simulink model "IEEE123_4subsystem"  (R2022b)
settings: Solver=ode4  StartTime=0.0  StopTime=inf  FixedStep=Ts  MaxStep=1e-4  RelTol=1e-3
PreLoadFcn:
  | Ts = 50e-6;
PostLoadFcn:
  | Ts = 50e-6;
InitFcn:
  | %%%%%%%%%%%%%%%%%%%%%%%%
  | % Simulation data for the IEEE 123 Node Test Feeder model
  | %%%%%%%%%%%%%%%%%%%%%%%
  | 
  | % miles/km
  | mi2km = 1.60934;
  | 
  | % feet to km
  | ft2km = 0.0003048;
  | 
  | % microsiemens to Farads
  | ms2F = 1/2/pi/60*1e-6;
  | 
  | %% Configuration 1 - series reactance - ohm/mile
  | 
  | R_1 = [0.4576 0.1560 0.1535;0.1560 0.4666 0.1580;0.1535 0.1580 0.4615];
  | X_1 = [1.0780 0.5017 0.3849;0.5017 1.0482 0.4236;0.3849 0.4236 1.0651];
  | 
  | % charging susceptance - microsiemens/mile
  | 
  | B_1 = [5.6765 -1.8319 -0.6982;-1.8319 5.9809 -1.1645;-0.6982 -1.1645 5.3971];
  | 
  | % convert for SPS
  | 
  | R_1 = R_1/mi2km;
  | 
  | Rs_1=(R_1(1,1)+R_1(2,2)+R_1(3,3))/3;
  | Rm_1=(R_1(1,2)+R_1(1,3)+R_1(2,3))/3;
  | R1_1=Rs_1-Rm_1;
  | R0_1=Rs_1+2*Rm_1;
  | 
  | L_1 = X_1/mi2km/2/pi/60;
  | 
  | Ls_1=(L_1(1,1)+L_1(2,2)+L_1(3,3))/3;
  | Lm_1=(L_1(1,2)+L_1(1,3)+L_1(2,3))/3;
  | L1_1=Ls_1-Lm_1;
  | L0_1=Ls_1+2*Lm_1;
  | 
  | C_1 = B_1/mi2km*ms2F;
  | 
  | Cs_1=(C_1(1,1)+C_1(2,2)+C_1(3,3))/3;
  | Cm_1=(C_1(1,2)+C_1(1,3)+C_1(2,3))/3;
  | C1_1=Cs_1-Cm_1;
  | C0_1=Cs_1+2*Cm_1;
  | 
  | 
  | %% Configuration 2 - series reactance - ohm/mile
  | 
  | R_2 = [0.4666 0.1580 0.1560;0.1580 0.4615 0.1535;0.1560 0.1535 0.4576];
  | X_2 = [1.0482 0.4236 0.5017;0.4236 1.0651 0.3849;0.5017 0.3849 1.0780];
  | 
  | % charging susceptance - microsiemens/mile
  | 
  | B_2 = [5.9809 -1.1645 -1.8319;-1.1645 5.3971 -0.6982;-1.8319 -0.6982 5.6765];
  | 
  | % convert for SPS
  | 
  | R_2 = R_2/mi2km;
  | 
  | Rs_2=(R_2(1,1)+R_2(2,2)+R_2(3,3))/3;
  | ... (+341 lines)
undefined symbols (not defined in the file): D1, Delta, find_system, I, Left, MOV_segment9, powergui, Right, type, V, X
libraries: spsGroundLib x242, spsThreePhaseVIMeasurementLib x134, spsSeriesRLCBranchLib x107, spsSeriesRLCLoadLib x83, spsPiSectionLineLib x61, spsThreePhasePISectionLineLib x60, spsVoltageMeasurementLib x52, spsDCVoltageSourceLib x36, ssn_lib x28, artemis x24, spsACCurrentSourceLib x18, spsOnDelayLib x18
(part 8 of 15)

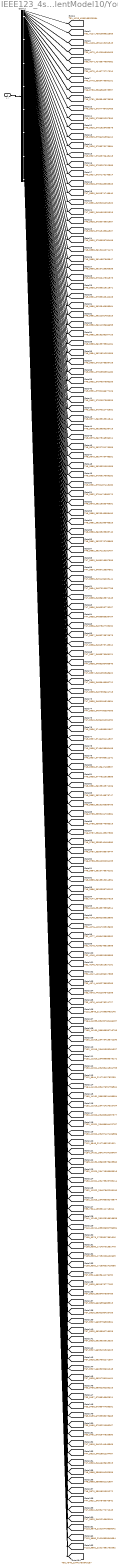
== system IEEE123_4subsystem/powergui/EquivalentModel10/Yout ==
  v,i : Inport
  Demux : Demux  Outputs=[1 1 1 1 1 1 1 1 1 1 1 1 1 1 1 1 1 1 1 1 1 1 1 1 1 1 1 1 1 1 1 1 1 1 1 1 1 1 1 1 1 1 1 1 1 1 1 1 1 1 1 1 1 1 1 1 1 1 1 1 1 1 1 1 1 1 1 1 1 1 1 1 1 1 1 1 1 1 1 1 1 1 1 1 1 1 1 1 1 1 1 1 1 1 1 1 1 1 1 1 1 1 1 1 1 1 1 1 1 1 1 1 1 1 1 1 1 1 1 1 1 1 1 1 1 1 1 1 1 1 1 1 1 1 1 1 1 1 1 1 1 1 1 1 1 1 1 1 1 1 1 1 1 1 1 1 1 1 1 1 1 1 1 1]
  tag scope: T109_9379_17239517861616=global, T109_9380_17245701551478=global, T109_9381_17252206402625=global, T109_9382_17259032415056=global, T112_9843_21170965463146=global, T112_9844_21171312782239=global, T112_9845_21171852131511=global, T113_9879_21016479838042=global, T113_9880_21016835649654=global, T113_9881_21017381792062=global, T132_11318_25473415572290=global, T132_11319_25472424310754=global, T132_11319_25481353264337=global, T132_11320_25471595983916=global, T132_11320_25480360057377=global, T132_11320_25489689575172=global, T132_11321_25479529785114=global, T132_11321_25488694422787=global, T132_11321_25498424504795=global, T132_11322_25487862205100=global, T132_11322_25497427406986=global, T132_11323_25496593243874=global, T141_12160_28102518618639=global, T142_12211_28300682796084=global, T164_14099_38430760466187=global, T164_14100_38427691756561=global, T164_14101_38424754189497=global, T165_14150_38606899716706=global, T165_14151_38603824498954=global, T165_14152_38600879628960=global, T46_3779_3365479900101=global, T46_3780_3366960378957=global, T46_3781_3368545675638=global, T46_3785_3359104702884=global, T46_3786_3358240484580=global, T46_3786_3360574906319=global, T46_3787_3359708975444=global, T46_3787_3362149927580=global, T46_3788_3361282284135=global, T47_3818_3461244945569=global, T47_3819_3462881234487=global, T47_3820_3464625615319=global, T47_3821_3457845970842=global, T47_3822_3459477271045=global, T47_3823_3461216663164=global, T47_3830_3491574748640=global, T47_3831_3493184294320=global, T47_3832_3494901931915=global, T47_3833_3488118997595=global, T47_3834_3487013057798=global, T47_3834_3489723554561=global, T47_3835_3485966639704=global, T47_3835_3488615871045=global, T47_3835_3491436203441=global, T47_3836_3484979743312=global, T47_3836_3487567709232=global, T47_3836_3490326776207=global, T47_3837_3484052368622=global, T47_3837_3486579069121=global, T47_3837_3489276870675=global, T47_3838_3483184515634=global, T47_3838_3485649950712=global, T47_3838_3488286486846=global, T47_3839_3484780354006=global, T47_3839_3487355624718=global, T47_3840_3486484284292=global, T48_3868_3588184282939=global, T48_3869_3589952131897=global, T48_3870_3591831351272=global, T48_3877_3623913311844=global, T48_3878_3622731176059=global, T48_3878_3625659238719=global, T48_3879_3621603340691=global, T48_3879_3624475448351=global, T48_3879_3627516536011=global, T48_3880_3620529805740=global, T48_3880_3620540608364=global, T48_3880_3623345958400=global, T48_3880_3626331091059=global, T48_3881_3619510571206=global, T48_3881_3622270768865=global, T48_3881_3622281452323=global, T48_3881_3625199946525=global, T48_3882_3618238287726=global, T48_3882_3621249879747=global, T48_3882_3624123102407=global, T48_3882_3624133666698=global, T48_3883_3619975584184=global, T48_3883_3623100558706=global, T48_3884_3616778670102=global, T48_3884_3621824251059=global, T48_3885_3618513014894=global, T48_3886_3620358730102=global, T48_3888_3613161071472=global, T48_3889_3614887665847=global, T48_3890_3616725630638=global, T49_3924_3757748792483=global, T49_3925_3756494356412=global, T49_3925_3759631297500=global, T49_3926_3755297012585=global, T49_3926_3758375175884=global, T49_3926_3761628455578=global, T49_3927_3757176146514=global, T49_3927_3760370648418=global, T49_3928_3753073601667=global, T49_3928_3759169933503=global, T49_3929_3752047534575=global, T49_3929_3754949364507=global, T49_3930_3750614909252=global, T49_3930_3751078559728=global, T49_3930_3753921611871=global, T49_3930_3756939780408=global, T49_3931_3750166677126=global, T49_3931_3752487418180=global, T49_3931_3752950951480=global, T49_3931_3755910342228=global, T49_3932_3752037383333=global, T49_3932_3754474580170=global, T49_3932_3754937996293=global, T49_3933_3754022742602=global, T49_3936_3744588901667=global, T49_3937_3743786611241=global, T49_3937_3746451414507=global, T49_3938_3745647438537=global, T49_3938_3748428580408=global, T49_3939_3747622918895=global, T50_4073_4242094590453=global, T50_4074_4243874684082=global, T50_4075_4245772717310=global, T50_4147_3946663207629=global, T50_4148_3948375596914=global, T50_4149_3950205925800=global, T51_4126_4390185320384=global, T51_4127_4392089622565=global, T51_4128_4394115154549=global, T51_4276_4184720319600=global, T51_4277_4186423803302=global, T51_4278_4188248516808=global, T52_4245_4199931959955=global, T52_4246_4201921827191=global, T52_4247_4204036217888=global, T53_4374_4430278693266=global, T53_4375_4432264542308=global, T53_4376_4434378211727=global, T63_5456_6800230253216=global, T63_5457_6799516962811=global, T63_5458_6798947459391=global, T63_5459_6793938078669=global, T63_5460_6793221056267=global, T63_5461_6792647820850=global, T67_5524_6628644176192=global, T67_5525_6626590718028=global, T67_5525_6626956688313=global, T67_5525_6631975777182=global, T67_5526_6624902271307=global, T67_5526_6629920913320=global, T67_5526_6630286426753=global, T67_5526_6635487595785=global, T67_5527_6628230604048=global, T67_5527_6633431326223=global, T67_5527_6633796382804=global, T67_5528_6631739154401=global, T89_7904_13533111748011=global, T90_7940_13442750943157=global
  wires:
  v,i/1 -> Demux/1
  Demux/1 -> [T51_4126_4390185320384]
  Demux/2 -> [T51_4127_4392089622565]
  Demux/3 -> [T51_4128_4394115154549]
  Demux/4 -> [T50_4073_4242094590453]
  Demux/5 -> [T50_4074_4243874684082]
  Demux/6 -> [T50_4075_4245772717310]
  Demux/7 -> [T46_3779_3365479900101]
  Demux/8 -> [T46_3780_3366960378957]
  Demux/9 -> [T46_3781_3368545675638]
  Demux/10 -> [T49_3924_3757748792483]
  Demux/11 -> [T49_3925_3759631297500]
  Demux/12 -> [T49_3926_3761628455578]
  Demux/13 -> [T49_3925_3756494356412]
  Demux/14 -> [T49_3926_3758375175884]
  Demux/15 -> [T49_3927_3760370648418]
  Demux/16 -> [T49_3926_3755297012585]
  Demux/17 -> [T49_3927_3757176146514]
  Demux/18 -> [T49_3928_3759169933503]
  Demux/19 -> [T47_3830_3491574748640]
  Demux/20 -> [T47_3831_3493184294320]
  Demux/21 -> [T47_3832_3494901931915]
  Demux/22 -> [T49_3928_3753073601667]
  Demux/23 -> [T49_3929_3754949364507]
  Demux/24 -> [T49_3930_3756939780408]
  Demux/25 -> [T48_3888_3613161071472]
  Demux/26 -> [T48_3889_3614887665847]
  Demux/27 -> [T48_3890_3616725630638]
  Demux/28 -> [T49_3929_3752047534575]
  Demux/29 -> [T49_3930_3753921611871]
  Demux/30 -> [T49_3931_3755910342228]
  Demux/31 -> [T48_3880_3620540608364]
  Demux/32 -> [T48_3881_3622281452323]
  Demux/33 -> [T48_3882_3624133666698]
  Demux/34 -> [T48_3882_3618238287726]
  Demux/35 -> [T48_3883_3619975584184]
  Demux/36 -> [T48_3884_3621824251059]
  Demux/37 -> [T49_3930_3751078559728]
  Demux/38 -> [T49_3931_3752950951480]
  Demux/39 -> [T49_3932_3754937996293]
  Demux/40 -> [T49_3931_3750166677126]
  Demux/41 -> [T49_3932_3752037383333]
  Demux/42 -> [T49_3933_3754022742602]
  Demux/43 -> [T48_3877_3623913311844]
  Demux/44 -> [T48_3878_3625659238719]
  Demux/45 -> [T48_3879_3627516536011]
  Demux/46 -> [T48_3878_3622731176059]
  Demux/47 -> [T48_3879_3624475448351]
  Demux/48 -> [T48_3880_3626331091059]
  Demux/49 -> [T49_3930_3750614909252]
  Demux/50 -> [T49_3931_3752487418180]
  Demux/51 -> [T49_3932_3754474580170]
  Demux/52 -> [T48_3879_3621603340691]
  Demux/53 -> [T48_3880_3623345958400]
  Demux/54 -> [T48_3881_3625199946525]
  Demux/55 -> [T48_3880_3620529805740]
  Demux/56 -> [T48_3881_3622270768865]
  Demux/57 -> [T48_3882_3624123102407]
  Demux/58 -> [T47_3833_3488118997595]
  Demux/59 -> [T47_3834_3489723554561]
  Demux/60 -> [T47_3835_3491436203441]
  Demux/61 -> [T47_3834_3487013057798]
  Demux/62 -> [T47_3835_3488615871045]
  Demux/63 -> [T47_3836_3490326776207]
  Demux/64 -> [T47_3835_3485966639704]
  Demux/65 -> [T47_3836_3487567709232]
  Demux/66 -> [T47_3837_3489276870675]
  Demux/67 -> [T47_3836_3484979743312]
  Demux/68 -> [T47_3837_3486579069121]
  Demux/69 -> [T47_3838_3488286486846]
  Demux/70 -> [T47_3837_3484052368622]
  Demux/71 -> [T47_3838_3485649950712]
  Demux/72 -> [T47_3839_3487355624718]
  Demux/73 -> [T47_3838_3483184515634]
  Demux/74 -> [T47_3839_3484780354006]
  Demux/75 -> [T47_3840_3486484284292]
  Demux/76 -> [T49_3936_3744588901667]
  Demux/77 -> [T49_3937_3746451414507]
  Demux/78 -> [T49_3938_3748428580408]
  Demux/79 -> [T49_3937_3743786611241]
  Demux/80 -> [T49_3938_3745647438537]
  Demux/81 -> [T49_3939_3747622918895]
  Demux/82 -> [T48_3881_3619510571206]
  Demux/83 -> [T48_3882_3621249879747]
  Demux/84 -> [T48_3883_3623100558706]
  Demux/85 -> [T46_3785_3359104702884]
  Demux/86 -> [T46_3786_3360574906319]
  Demux/87 -> [T46_3787_3362149927580]
  Demux/88 -> [T46_3786_3358240484580]
  Demux/89 -> [T46_3787_3359708975444]
  Demux/90 -> [T46_3788_3361282284135]
  Demux/91 -> [T48_3884_3616778670102]
  Demux/92 -> [T48_3885_3618513014894]
  Demux/93 -> [T48_3886_3620358730102]
  Demux/94 -> [T50_4147_3946663207629]
  Demux/95 -> [T50_4148_3948375596914]
  Demux/96 -> [T50_4149_3950205925800]
  Demux/97 -> [T51_4276_4184720319600]
  Demux/98 -> [T51_4277_4186423803302]
  Demux/99 -> [T51_4278_4188248516808]
  Demux/100 -> [T52_4245_4199931959955]
  Demux/101 -> [T52_4246_4201921827191]
  Demux/102 -> [T52_4247_4204036217888]
  Demux/103 -> [T53_4374_4430278693266]
  Demux/104 -> [T53_4375_4432264542308]
  Demux/105 -> [T53_4376_4434378211727]
  Demux/106 -> [T112_9843_21170965463146]
  Demux/107 -> [T164_14099_38430760466187]
  Demux/108 -> [T165_14150_38606899716706]
  Demux/109 -> [T132_11318_25473415572290]
  Demux/110 -> [T132_11319_25481353264337]
  Demux/111 -> [T132_11320_25489689575172]
  Demux/112 -> [T132_11321_25498424504795]
  Demux/113 -> [T112_9844_21171312782239]
  Demux/114 -> [T164_14100_38427691756561]
  Demux/115 -> [T165_14151_38603824498954]
  Demux/116 -> [T132_11319_25472424310754]
  Demux/117 -> [T132_11320_25480360057377]
  Demux/118 -> [T132_11321_25488694422787]
  Demux/119 -> [T132_11322_25497427406986]
  Demux/120 -> [T112_9845_21171852131511]
  Demux/121 -> [T164_14101_38424754189497]
  Demux/122 -> [T165_14152_38600879628960]
  Demux/123 -> [T132_11320_25471595983916]
  Demux/124 -> [T132_11321_25479529785114]
  Demux/125 -> [T132_11322_25487862205100]
  Demux/126 -> [T132_11323_25496593243874]
  Demux/127 -> [T89_7904_13533111748011]
  Demux/128 -> [T141_12160_28102518618639]
  Demux/129 -> [T142_12211_28300682796084]
  Demux/130 -> [T109_9379_17239517861616]
  Demux/131 -> [T109_9380_17245701551478]
  Demux/132 -> [T109_9381_17252206402625]
  Demux/133 -> [T109_9382_17259032415056]
  Demux/134 -> [T67_5524_6628644176192]
  Demux/135 -> [T67_5525_6631975777182]
  Demux/136 -> [T67_5526_6635487595785]
  Demux/137 -> [T67_5525_6626956688313]
  Demux/138 -> [T67_5526_6630286426753]
  Demux/139 -> [T67_5527_6633796382804]
  Demux/140 -> [T67_5525_6626590718028]
  Demux/141 -> [T67_5526_6629920913320]
  Demux/142 -> [T67_5527_6633431326223]
  Demux/143 -> [T67_5526_6624902271307]
  Demux/144 -> [T67_5527_6628230604048]
  Demux/145 -> [T67_5528_6631739154401]
  Demux/146 -> [T63_5456_6800230253216]
  Demux/147 -> [T63_5457_6799516962811]
  Demux/148 -> [T63_5458_6798947459391]
  Demux/149 -> [T63_5459_6793938078669]
  Demux/150 -> [T63_5460_6793221056267]
  Demux/151 -> [T63_5461_6792647820850]
  Demux/152 -> [T47_3818_3461244945569]
  Demux/153 -> [T47_3819_3462881234487]
  Demux/154 -> [T47_3820_3464625615319]
  Demux/155 -> [T48_3868_3588184282939]
  Demux/156 -> [T48_3869_3589952131897]
  Demux/157 -> [T48_3870_3591831351272]
  Demux/158 -> [T47_3821_3457845970842]
  Demux/159 -> [T47_3822_3459477271045]
  Demux/160 -> [T47_3823_3461216663164]
  Demux/161 -> [T113_9879_21016479838042]
  Demux/162 -> [T113_9880_21016835649654]
  Demux/163 -> [T113_9881_21017381792062]
  Demux/164 -> [T90_7940_13442750943157]

== system IEEE123_4subsystem/powergui/EquivalentModel11/Gates ==
  Mux : Mux  Inputs=[1 1 1 1 1 1 1 1 1]
  gates : Outport  VectorParamsAs1DForOutWhenUnconnected=off
  wires:
  Mux/1 -> gates/1
  [T47_3746_3326232538788] -> Mux/1
  [T47_3747_3328761381711] -> Mux/2
  [T47_3748_3331415692294] -> Mux/3
  [T49_3849_3558680962917] -> Mux/4
  [T49_3850_3561486331293] -> Mux/5
  [T49_3851_3564423847015] -> Mux/6
  [T47_3756_3318374942812] -> Mux/7
  [T47_3757_3320884542137] -> Mux/8
  [T47_3758_3323519609121] -> Mux/9

== system IEEE123_4subsystem/powergui/EquivalentModel11/Sources ==
  Mux : Mux  Inputs=[1 1 1 1 1 1 1 1 1 1 1 1 1 1 1 1 1 1 1 1 1 1 1 1 1 1 1 1 1 1 1 1 1 1 1 1 1 1 1 1 1 1 1 1 1 1 1 1 1 1 1 1 1 1 1 1 1 1 1 1 1 1 1 1 1 1 1 1 1 1 1 1]
  Mux_u : Mux  Inputs=[9 72]
  SwitchCurrents : Constant  Value=zeros(9,1)
  u : Outport  VectorParamsAs1DForOutWhenUnconnected=off
  wires:
  Mux_u/1 -> u/1
  SwitchCurrents/1 -> Mux_u/1
  Mux/1 -> Mux_u/2
  [T149_12763_31024626200921] -> Mux/1
  [T150_12814_31269076500165] -> Mux/2
  [T119_10174_20208376729007] -> Mux/3
  [T119_10176_20232093387237] -> Mux/4
  [T119_10178_20256488954274] -> Mux/5
  [T119_10180_20281563430120] -> Mux/6
  [T149_12764_31021204114740] -> Mux/7
  [T150_12815_31265654163596] -> Mux/8
  [T119_10175_20206177324800] -> Mux/9
  [T119_10177_20229890930254] -> Mux/10
  [T119_10179_20254283444515] -> Mux/11
  [T119_10181_20279354867584] -> Mux/12
  [T149_12765_31017857733390] -> Mux/13
  [T150_12816_31262307027159] -> Mux/14
  [T119_10176_20204072710677] -> Mux/15
  [T119_10178_20227783263354] -> Mux/16
  [T119_10180_20252172724840] -> Mux/17
  [T119_10182_20277241095133] -> Mux/18
  [T76_6173_8376833568932] -> Mux/19
  [T76_6174_8381053757100] -> Mux/20
  [T76_6175_8385484270532] -> Mux/21
  [T76_6174_8374857078672] -> Mux/22
  [T76_6175_8379075522756] -> Mux/23
  [T76_6176_8383504292104] -> Mux/24
  [T75_6132_8111398398198] -> Mux/25
  [T75_6133_8115484561917] -> Mux/26
  [T75_6134_8119777701903] -> Mux/27
  [T75_6133_8109393145182] -> Mux/28
  [T75_6134_8113477584998] -> Mux/29
  [T75_6135_8117769001081] -> Mux/30
  [T75_6133_8109477733885] -> Mux/31
  [T75_6134_8113562586422] -> Mux/32
  [T75_6135_8117854415225] -> Mux/33
  [T75_6134_8107471672728] -> Mux/34
  [T75_6135_8111554801362] -> Mux/35
  [T75_6136_8115844906263] -> Mux/36
  [T105_8930_15251430888447] -> Mux/37
  [T105_8931_15258125161535] -> Mux/38
  [T105_8931_15250142436535] -> Mux/39
  [T105_8932_15256834925654] -> Mux/40
  [T105_8932_15248961413385] -> Mux/41
  [T105_8933_15255652118535] -> Mux/42
  [T84_7398_12385968697709] -> Mux/43
  [T84_7399_12383315155818] -> Mux/44
  [T84_7400_12380769454164] -> Mux/45
  [T84_7403_12372177511664] -> Mux/46
  [T84_7404_12369520384686] -> Mux/47
  [T84_7405_12366971097946] -> Mux/48
  [T137_11711_25482651457792] -> Mux/49
  [T138_11762_25623014118441] -> Mux/50
  [T137_11712_25479701659419] -> Mux/51
  [T138_11763_25620063700182] -> Mux/52
  [T137_11713_25476834196959] -> Mux/53
  [T138_11764_25617195021198] -> Mux/54
  [T64_5121_5460278169621] -> Mux/55
  [T64_5122_5464275454759] -> Mux/56
  [T64_5123_5468455144898] -> Mux/57
  [T64_5122_5459212516744] -> Mux/58
  [T64_5123_5463207694819] -> Mux/59
  [T64_5124_5467385277894] -> Mux/60
  [T63_5080_5265999666590] -> Mux/61
  [T63_5081_5269850985320] -> Mux/62
  [T63_5082_5273881351987] -> Mux/63
  [T63_5081_5264876398940] -> Mux/64
  [T63_5082_5268725629636] -> Mux/65
  [T63_5083_5272753908269] -> Mux/66
  [T63_5081_5264673306411] -> Mux/67
  [T63_5082_5268523037005] -> Mux/68
  [T63_5083_5272551815535] -> Mux/69
  [T63_5082_5263548890481] -> Mux/70
  [T63_5083_5267396533041] -> Mux/71
  [T63_5084_5271423223538] -> Mux/72

== system IEEE123_4subsystem/powergui/EquivalentModel11/State-Space ==
  In1 : Inport
  In2 : Inport  Port=2
  ssn_sfun_sw1 : S-Function  FunctionName=ssn_sfun_v1  Parameters=11,0  SFunctionDeploymentMode=off  EnableBusSupport=off  SFcnStateName=MOV_segment79,xn_g1,xn_g2,xn_g3,xn_g4,xn_g5,xn_g6,xn_g7,MOV_segment79,MOV_segment79,MOV_segment79,MOV_segment79,MOV_segment79,MOV_segment79,MOV_segment79,MOV_segment79,MOV_segment79,MOV_segment79,MOV_segment79,MOV_segment79,MOV_segment79,MOV_segment79,MOV_segment79,MOV_segment79,MOV_segment79,MOV_segment79,MOV_segment79,MOV_segment79,MOV_segment79,MOV_segment79,MOV_segment79,MOV_segment79,MOV_segment79,MOV_segment79,MOV_segment79,MOV_segment79,MOV_segment79,MOV_segment79,MOV_segment79,MOV_segment79,MOV_segment79,MOV_segment79,MOV_segment79,MOV_segment79,MOV_segment79,MOV_segment79,MOV_segment79,MOV_segment79,MOV_segment79,MOV_segment79,MOV_segment79,MOV_segment79,MOV_segment79,MOV_segment79,MOV_segment79,MOV_segment79,MOV_segment79,MOV_segment79,MOV_segment79,MOV_segment79,MOV_segment79,MOV_segment79,MOV_segment79,MOV_segment79,MOV_segment79,MOV_segment79,MOV_segment79,MOV_segment79,MOV_segment79,MOV_segment79,MOV_segment79,MOV_segment79,MOV_segment79,MOV_segment79,MOV_segment79,MOV_segment79,MOV_segment79,MOV_segment79,MOV_segment79,MOV_segment79
      settings: SFcnIsStateOwnerBlock=on
  Out1 : Outport  VectorParamsAs1DForOutWhenUnconnected=off
  Out2 : Outport  Port=2  VectorParamsAs1DForOutWhenUnconnected=off
  tag scope: ssn_ext_sys_from_V_0bexa56ax8042611b062e=global, ssn_ext_sys_from_V_28dxbbddxddcdb436b4ad=global, ssn_ext_sys_from_V_eecxba08x8fb44e0fabb4=global
  wires:
  ssn_sfun_sw1/2 -> Out2/1
  In2/1 -> ssn_sfun_sw1/2
  ssn_sfun_sw1/1 -> Out1/1
  In1/1 -> ssn_sfun_sw1/1
  [ssn_ext_sys_goto_Hist_0bexa56ax8042611b062e] -> ssn_sfun_sw1/3
  [ssn_ext_sys_goto_Y_0bexa56ax8042611b062e] -> ssn_sfun_sw1/4
  ssn_sfun_sw1/3 -> [ssn_ext_sys_from_V_0bexa56ax8042611b062e]
  [ssn_ext_sys_goto_Hist_28dxbbddxddcdb436b4ad] -> ssn_sfun_sw1/5
  [ssn_ext_sys_goto_Y_28dxbbddxddcdb436b4ad] -> ssn_sfun_sw1/6
  ssn_sfun_sw1/4 -> [ssn_ext_sys_from_V_28dxbbddxddcdb436b4ad]
  [ssn_ext_sys_goto_Hist_eecxba08x8fb44e0fabb4] -> ssn_sfun_sw1/7
  [ssn_ext_sys_goto_Y_eecxba08x8fb44e0fabb4] -> ssn_sfun_sw1/8
  ssn_sfun_sw1/5 -> [ssn_ext_sys_from_V_eecxba08x8fb44e0fabb4]

== system IEEE123_4subsystem/powergui/EquivalentModel11/Status ==
  status : Inport
  Demux : Demux  Outputs=[1 1 1 1 1 1 1 1 1]
  tag scope: T49_3981_4083145854575=global, T49_3982_4085119922764=global, T49_3983_4087214337483=global, T49_3991_4072447264371=global, T49_3992_4074403643503=global, T49_3993_4076480369167=global, T51_4084_4368197134149=global, T51_4085_4370433853067=global, T51_4086_4372797537082=global
  wires:
  status/1 -> Demux/1
  Demux/1 -> [T49_3981_4083145854575]
  Demux/2 -> [T49_3982_4085119922764]
  Demux/3 -> [T49_3983_4087214337483]
  Demux/4 -> [T51_4084_4368197134149]
  Demux/5 -> [T51_4085_4370433853067]
  Demux/6 -> [T51_4086_4372797537082]
  Demux/7 -> [T49_3991_4072447264371]
  Demux/8 -> [T49_3992_4074403643503]
  Demux/9 -> [T49_3993_4076480369167]

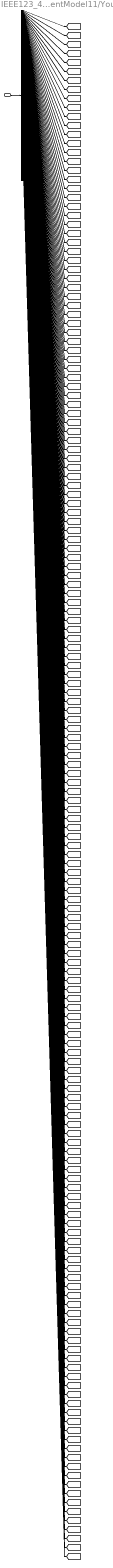
== system IEEE123_4subsystem/powergui/EquivalentModel11/Yout ==
  v,i : Inport
  Demux : Demux  Outputs=[1 1 1 1 1 1 1 1 1 1 1 1 1 1 1 1 1 1 1 1 1 1 1 1 1 1 1 1 1 1 1 1 1 1 1 1 1 1 1 1 1 1 1 1 1 1 1 1 1 1 1 1 1 1 1 1 1 1 1 1 1 1 1 1 1 1 1 1 1 1 1 1 1 1 1 1 1 1 1 1 1 1 1 1 1 1 1 1 1 1 1 1 1 1 1 1 1 1 1 1 1 1 1 1 1 1 1 1 1 1 1 1 1 1 1 1 1 1 1 1 1 1 1 1 1 1 1 1 1 1 1 1 1 1 1 1 1 1 1 1 1 1 1 1 1 1 1 1 1 1 1 1 1 1 1 1 1 1 1 1 1 1 1 1 1 1 1 1 1 1 1]
  tag scope: T110_9436_17627002952868=global, T110_9437_17625253054596=global, T110_9437_17633282360121=global, T110_9438_17623605701959=global, T110_9438_17631530788227=global, T110_9438_17639886293919=global, T110_9439_17629881761969=global, T110_9439_17638133048404=global, T110_9439_17646814754263=global, T110_9440_17636482348525=global, T110_9440_17645059835126=global, T110_9441_17643407461626=global, T142_12217_28588295635819=global, T142_12218_28585047524811=global, T142_12219_28581878850563=global, T143_12268_28785342288521=global, T143_12269_28782094359608=global, T143_12270_28778925311954=global, T48_3875_3584240296981=global, T48_3876_3585999125940=global, T48_3877_3587869325315=global, T48_3880_3579019836809=global, T48_3881_3580769797017=global, T48_3882_3582631127642=global, T48_3885_3574897900638=global, T48_3886_3574161977939=global, T48_3886_3576639170847=global, T48_3887_3575901474397=global, T48_3887_3578491811472=global, T48_3887_3616493825811=global, T48_3888_3577752341272=global, T48_3888_3615304711702=global, T48_3888_3618225649770=global, T48_3889_3614178001343=global, T48_3889_3617034761910=global, T48_3889_3620068844145=global, T48_3890_3613113694734=global, T48_3890_3615906277801=global, T48_3890_3618876182535=global, T48_3891_3612111791875=global, T48_3891_3614840197442=global, T48_3891_3617745924676=global, T48_3892_3611172292766=global, T48_3892_3613836520833=global, T48_3892_3616678070567=global, T48_3893_3610295197407=global, T48_3893_3612895247974=global, T48_3893_3615672620208=global, T48_3894_3612016378865=global, T48_3894_3614729573599=global, T48_3895_3613848930740=global, T48_3897_3606951320851=global, T48_3898_3606195183577=global, T48_3898_3608665586059=global, T48_3899_3605501450053=global, T48_3899_3607907675035=global, T48_3899_3610491221684=global, T48_3900_3607212167762=global, T48_3900_3609731536910=global, T48_3901_3609034255887=global, T49_3930_3754241613027=global, T49_3931_3753104803503=global, T49_3931_3756117109966=global, T49_3932_3751896505816=global, T49_3932_3754978497721=global, T49_3932_3758107259966=global, T49_3933_3753768631667=global, T49_3933_3756966845000=global, T49_3934_3755755410578=global, T49_3935_3749210626633=global, T49_3936_3747949506395=global, T49_3936_3751077109966=global, T49_3937_3749814538537=global, T49_3937_3753058246361=global, T49_3938_3745394881395=global, T49_3938_3746975708265=global, T49_3938_3751794223741=global, T49_3939_3747256601037=global, T49_3939_3748836783435=global, T49_3940_3749232973741=global, T49_3940_3750812511667=global, T49_3946_3738959544167=global, T49_3947_3740806724864=global, T49_3948_3742768558622=global, T49_3992_3735120557789=global, T49_3993_3736890144864=global, T49_3994_3738774385000=global, T50_4002_3830720087024=global, T50_4003_3832346289388=global, T50_4004_3834555517894=global, T50_4080_4236941146633=global, T50_4081_4238712516800=global, T50_4082_4240601826567=global, T50_4090_4225316094873=global, T50_4091_4227070483547=global, T50_4092_4228942811820=global, T51_4028_4021198610565=global, T51_4029_4020017653702=global, T51_4029_4020140852949=global, T51_4029_4023341543584=global, T51_4030_4018899441937=global, T51_4030_4019086600400=global, T51_4030_4022158842408=global, T51_4030_4022281984965=global, T51_4030_4025605706408=global, T51_4031_4017843975271=global, T51_4031_4018095092949=global, T51_4031_4021038886329=global, T51_4031_4021225988102=global, T51_4031_4024421260918=global, T51_4031_4024544346784=global, T51_4032_4016851253702=global, T51_4032_4019981675349=global, T51_4032_4020232736337=global, T51_4032_4023299560525=global, T51_4032_4023486605608=global, T51_4033_4016300313341=global, T51_4033_4018987209467=global, T51_4033_4022240605231=global, T51_4033_4022491609529=global, T51_4034_4015497041184=global, T51_4034_4018434468102=global, T51_4034_4021244395035=global, T51_4035_4017629451631=global, T51_4035_4020689852667=global, T51_4036_4014078732165=global, T51_4036_4019883091882=global, T51_4037_4016207653984=global, T51_4038_4018457805608=global, T51_4193_4057059134141=global, T51_4194_4058915956102=global, T51_4195_4060894007867=global, T51_4205_4092024169435=global, T51_4206_4093853256808=global, T51_4207_4095803573984=global, T52_4183_4537107975577=global, T52_4184_4539135145354=global, T52_4185_4541286838594=global, T52_4334_4342598604446=global, T52_4335_4344417132308=global, T52_4336_4346360183631=global, T63_5455_6802410388223=global, T63_5456_6801698341818=global, T63_5457_6801130082396=global, T63_5460_6791783722217=global, T63_5461_6791065276626=global, T63_5462_6790490618018=global, T68_5586_6831124591361=global, T68_5587_6829419723554=global, T68_5587_6829457372790=global, T68_5587_6834562599921=global, T68_5588_6827751520527=global, T68_5588_6832856299849=global, T68_5588_6832893498251=global, T68_5588_6838184167305=global, T68_5589_6831186213723=global, T68_5589_6836476434967=global, T68_5589_6836513182535=global, T68_5590_6834804465742=global, T69_5627_7067051836257=global, T69_5628_7065427953649=global, T69_5628_7070628136752=global, T69_5629_7069002351040=global, T69_5629_7074391338406=global, T69_5630_7072763649591=global, T90_7961_13892834698703=global, T90_7962_13892066965748=global, T90_7963_13891424566348=global, T91_7997_13798902114274=global, T91_7998_13798152165123=global, T91_7999_13797526172237=global
  wires:
  v,i/1 -> Demux/1
  Demux/1 -> [T50_4080_4236941146633]
  Demux/2 -> [T50_4081_4238712516800]
  Demux/3 -> [T50_4082_4240601826567]
  Demux/4 -> [T52_4183_4537107975577]
  Demux/5 -> [T52_4184_4539135145354]
  Demux/6 -> [T52_4185_4541286838594]
  Demux/7 -> [T50_4090_4225316094873]
  Demux/8 -> [T50_4091_4227070483547]
  Demux/9 -> [T50_4092_4228942811820]
  Demux/10 -> [T49_3930_3754241613027]
  Demux/11 -> [T49_3931_3756117109966]
  Demux/12 -> [T49_3932_3758107259966]
  Demux/13 -> [T49_3931_3753104803503]
  Demux/14 -> [T49_3932_3754978497721]
  Demux/15 -> [T49_3933_3756966845000]
  Demux/16 -> [T51_4029_4020140852949]
  Demux/17 -> [T51_4030_4022281984965]
  Demux/18 -> [T51_4031_4024544346784]
  Demux/19 -> [T51_4030_4019086600400]
  Demux/20 -> [T51_4031_4021225988102]
  Demux/21 -> [T51_4032_4023486605608]
  Demux/22 -> [T51_4031_4018095092949]
  Demux/23 -> [T51_4032_4020232736337]
  Demux/24 -> [T51_4033_4022491609529]
  Demux/25 -> [T49_3935_3749210626633]
  Demux/26 -> [T49_3936_3751077109966]
  Demux/27 -> [T49_3937_3753058246361]
  Demux/28 -> [T51_4033_4016300313341]
  Demux/29 -> [T51_4034_4018434468102]
  Demux/30 -> [T51_4035_4020689852667]
  Demux/31 -> [T51_4034_4015497041184]
  Demux/32 -> [T51_4035_4017629451631]
  Demux/33 -> [T51_4036_4019883091882]
  Demux/34 -> [T49_3938_3746975708265]
  Demux/35 -> [T49_3939_3748836783435]
  Demux/36 -> [T49_3940_3750812511667]
  Demux/37 -> [T51_4036_4014078732165]
  Demux/38 -> [T51_4037_4016207653984]
  Demux/39 -> [T51_4038_4018457805608]
  Demux/40 -> [T51_4028_4021198610565]
  Demux/41 -> [T51_4029_4023341543584]
  Demux/42 -> [T51_4030_4025605706408]
  Demux/43 -> [T51_4029_4020017653702]
  Demux/44 -> [T51_4030_4022158842408]
  Demux/45 -> [T51_4031_4024421260918]
  Demux/46 -> [T51_4030_4018899441937]
  Demux/47 -> [T51_4031_4021038886329]
  Demux/48 -> [T51_4032_4023299560525]
  Demux/49 -> [T51_4031_4017843975271]
  Demux/50 -> [T51_4032_4019981675349]
  Demux/51 -> [T51_4033_4022240605231]
  Demux/52 -> [T51_4032_4016851253702]
  Demux/53 -> [T51_4033_4018987209467]
  Demux/54 -> [T51_4034_4021244395035]
  Demux/55 -> [T49_3936_3747949506395]
  Demux/56 -> [T49_3937_3749814538537]
  Demux/57 -> [T49_3938_3751794223741]
  Demux/58 -> [T49_3946_3738959544167]
  Demux/59 -> [T49_3947_3740806724864]
  Demux/60 -> [T49_3948_3742768558622]
  Demux/61 -> [T49_3932_3751896505816]
  Demux/62 -> [T49_3933_3753768631667]
  Demux/63 -> [T49_3934_3755755410578]
  Demux/64 -> [T49_3938_3745394881395]
  Demux/65 -> [T49_3939_3747256601037]
  Demux/66 -> [T49_3940_3749232973741]
  Demux/67 -> [T48_3887_3616493825811]
  Demux/68 -> [T48_3888_3618225649770]
  Demux/69 -> [T48_3889_3620068844145]
  Demux/70 -> [T48_3888_3615304711702]
  Demux/71 -> [T48_3889_3617034761910]
  Demux/72 -> [T48_3890_3618876182535]
  Demux/73 -> [T50_4002_3830720087024]
  Demux/74 -> [T50_4004_3834555517894]
  Demux/75 -> [T50_4003_3832346289388]
  Demux/76 -> [T48_3889_3614178001343]
  Demux/77 -> [T48_3890_3615906277801]
  Demux/78 -> [T48_3891_3617745924676]
  Demux/79 -> [T48_3890_3613113694734]
  Demux/80 -> [T48_3891_3614840197442]
  Demux/81 -> [T48_3892_3616678070567]
  Demux/82 -> [T48_3891_3612111791875]
  Demux/83 -> [T48_3892_3613836520833]
  Demux/84 -> [T48_3893_3615672620208]
  Demux/85 -> [T48_3892_3611172292766]
  Demux/86 -> [T48_3893_3612895247974]
  Demux/87 -> [T48_3894_3614729573599]
  Demux/88 -> [T48_3893_3610295197407]
  Demux/89 -> [T48_3894_3612016378865]
  Demux/90 -> [T48_3895_3613848930740]
  Demux/91 -> [T48_3897_3606951320851]
  Demux/92 -> [T48_3898_3608665586059]
  Demux/93 -> [T48_3899_3610491221684]
  Demux/94 -> [T48_3898_3606195183577]
  Demux/95 -> [T48_3899_3607907675035]
  Demux/96 -> [T48_3900_3609731536910]
  Demux/97 -> [T48_3899_3605501450053]
  Demux/98 -> [T48_3900_3607212167762]
  Demux/99 -> [T48_3901_3609034255887]
  Demux/100 -> [T51_4205_4092024169435]
  Demux/101 -> [T51_4206_4093853256808]
  Demux/102 -> [T51_4207_4095803573984]
  Demux/103 -> [T52_4334_4342598604446]
  Demux/104 -> [T52_4335_4344417132308]
  Demux/105 -> [T52_4336_4346360183631]
  Demux/106 -> [T90_7961_13892834698703]
  Demux/107 -> [T142_12217_28588295635819]
  Demux/108 -> [T143_12268_28785342288521]
  Demux/109 -> [T110_9436_17627002952868]
  Demux/110 -> [T110_9437_17633282360121]
  Demux/111 -> [T110_9438_17639886293919]
  Demux/112 -> [T110_9439_17646814754263]
  Demux/113 -> [T90_7962_13892066965748]
  Demux/114 -> [T142_12218_28585047524811]
  Demux/115 -> [T143_12269_28782094359608]
  Demux/116 -> [T110_9437_17625253054596]
  Demux/117 -> [T110_9438_17631530788227]
  Demux/118 -> [T110_9439_17638133048404]
  Demux/119 -> [T110_9440_17645059835126]
  Demux/120 -> [T90_7963_13891424566348]
  Demux/121 -> [T142_12219_28581878850563]
  Demux/122 -> [T143_12270_28778925311954]
  Demux/123 -> [T110_9438_17623605701959]
  Demux/124 -> [T110_9439_17629881761969]
  Demux/125 -> [T110_9440_17636482348525]
  Demux/126 -> [T110_9441_17643407461626]
  Demux/127 -> [T69_5627_7067051836257]
  Demux/128 -> [T69_5628_7070628136752]
  Demux/129 -> [T69_5629_7074391338406]
  Demux/130 -> [T69_5628_7065427953649]
  Demux/131 -> [T69_5629_7069002351040]
  Demux/132 -> [T69_5630_7072763649591]
  Demux/133 -> [T68_5586_6831124591361]
  Demux/134 -> [T68_5587_6834562599921]
  Demux/135 -> [T68_5588_6838184167305]
  Demux/136 -> [T68_5587_6829457372790]
  Demux/137 -> [T68_5588_6832893498251]
  Demux/138 -> [T68_5589_6836513182535]
  Demux/139 -> [T68_5587_6829419723554]
  Demux/140 -> [T68_5588_6832856299849]
  Demux/141 -> [T68_5589_6836476434967]
  Demux/142 -> [T68_5588_6827751520527]
  Demux/143 -> [T68_5589_6831186213723]
  Demux/144 -> [T68_5590_6834804465742]
  Demux/145 -> [T49_3992_3735120557789]
  Demux/146 -> [T49_3993_3736890144864]
  Demux/147 -> [T49_3994_3738774385000]
  Demux/148 -> [T63_5455_6802410388223]
  Demux/149 -> [T63_5456_6801698341818]
  Demux/150 -> [T63_5457_6801130082396]
  Demux/151 -> [T63_5460_6791783722217]
  Demux/152 -> [T63_5461_6791065276626]
  Demux/153 -> [T63_5462_6790490618018]
  Demux/154 -> [T48_3875_3584240296981]
  Demux/155 -> [T48_3876_3585999125940]
  Demux/156 -> [T48_3877_3587869325315]
  Demux/157 -> [T48_3880_3579019836809]
  Demux/158 -> [T48_3881_3580769797017]
  Demux/159 -> [T48_3882_3582631127642]
  Demux/160 -> [T48_3885_3574897900638]
  Demux/161 -> [T48_3886_3576639170847]
  Demux/162 -> [T48_3887_3578491811472]
  Demux/163 -> [T48_3886_3574161977939]
  Demux/164 -> [T48_3887_3575901474397]
  Demux/165 -> [T48_3888_3577752341272]
  Demux/166 -> [T51_4193_4057059134141]
  Demux/167 -> [T51_4194_4058915956102]
  Demux/168 -> [T51_4195_4060894007867]
  Demux/169 -> [T91_7997_13798902114274]
  Demux/170 -> [T91_7998_13798152165123]
  Demux/171 -> [T91_7999_13797526172237]

== system IEEE123_4subsystem/powergui/EquivalentModel2/Sources ==
  Mux : Mux  Inputs=[1 1]
  u : Outport  VectorParamsAs1DForOutWhenUnconnected=off
  wires:
  Mux/1 -> u/1
  [T90_7740_12468903784605] -> Mux/1
  [T90_7727_12388780295467] -> Mux/2

== system IEEE123_4subsystem/powergui/EquivalentModel2/Yout ==
  v,i : Inport
  Demux : Demux  Outputs=1
  tag scope: T93_8272_15370932673394=global
  wires:
  v,i/1 -> Demux/1
  Demux/1 -> [T93_8272_15370932673394]

== system IEEE123_4subsystem/powergui/EquivalentModel3/Sources ==
  Mux : Mux  Inputs=[1 1]
  u : Outport  VectorParamsAs1DForOutWhenUnconnected=off
  wires:
  Mux/1 -> u/1
  [T91_7797_12800085321187] -> Mux/1
  [T91_7784_12718328472615] -> Mux/2

== system IEEE123_4subsystem/powergui/EquivalentModel3/Yout ==
  v,i : Inport
  Demux : Demux  Outputs=1
  tag scope: T94_8329_15750235785898=global
  wires:
  v,i/1 -> Demux/1
  Demux/1 -> [T94_8329_15750235785898]

== system IEEE123_4subsystem/powergui/EquivalentModel4/Sources ==
  Mux : Mux  Inputs=[1 1]
  u : Outport  VectorParamsAs1DForOutWhenUnconnected=off
  wires:
  Mux/1 -> u/1
  [T91_7798_12799685310527] -> Mux/1
  [T91_7785_12717953805226] -> Mux/2

== system IEEE123_4subsystem/powergui/EquivalentModel4/Yout ==
  v,i : Inport
  Demux : Demux  Outputs=1
  tag scope: T94_8330_15749048442184=global
  wires:
  v,i/1 -> Demux/1
  Demux/1 -> [T94_8330_15749048442184]

== system IEEE123_4subsystem/powergui/EquivalentModel5/Sources ==
  Mux : Mux  Inputs=[1 1]
  u : Outport  VectorParamsAs1DForOutWhenUnconnected=off
  wires:
  Mux/1 -> u/1
  [T91_7799_12799409256132] -> Mux/1
  [T91_7786_12717703094100] -> Mux/2

== system IEEE123_4subsystem/powergui/EquivalentModel5/Yout ==
  v,i : Inport
  Demux : Demux  Outputs=1
  tag scope: T94_8331_15747981098682=global
  wires:
  v,i/1 -> Demux/1
  Demux/1 -> [T94_8331_15747981098682]

== system IEEE123_4subsystem/powergui/EquivalentModel6/Sources ==
  Mux : Mux  Inputs=[1 1]
  u : Outport  VectorParamsAs1DForOutWhenUnconnected=off
  wires:
  Mux/1 -> u/1
  [T90_7765_12417060174976] -> Mux/1
  [T90_7752_12337521642017] -> Mux/2

== system IEEE123_4subsystem/powergui/EquivalentModel6/Yout ==
  v,i : Inport
  Demux : Demux  Outputs=1
  tag scope: T93_8297_15302327706914=global
  wires:
  v,i/1 -> Demux/1
  Demux/1 -> [T93_8297_15302327706914]

== system IEEE123_4subsystem/powergui/EquivalentModel7/Sources ==
  Mux : Mux  Inputs=[1 1]
  u : Outport  VectorParamsAs1DForOutWhenUnconnected=off
  wires:
  Mux/1 -> u/1
  [T90_7767_12416190864414] -> Mux/1
  [T90_7754_12336702637074] -> Mux/2

== system IEEE123_4subsystem/powergui/EquivalentModel7/Yout ==
  v,i : Inport
  Demux : Demux  Outputs=1
  tag scope: T93_8299_15299900970393=global
  wires:
  v,i/1 -> Demux/1
  Demux/1 -> [T93_8299_15299900970393]

== system IEEE123_4subsystem/powergui/EquivalentModel8/Sources ==
  Mux : Mux  Inputs=[1 1 1]
  u : Outport  VectorParamsAs1DForOutWhenUnconnected=off
  wires:
  Mux/1 -> u/1
  [T84_7399_12383059654727] -> Mux/1
  [T84_7400_12380405315506] -> Mux/2
  [T84_7401_12377858816523] -> Mux/3

== system IEEE123_4subsystem/powergui/EquivalentModel8/Yout ==
  v,i : Inport
  Demux : Demux  Outputs=[1 1 1 1 1 1 1 1 1 1 1 1 1 1 1 1 1 1 1 1 1 1 1 1 1 1 1 1 1 1 1 1 1 1 1 1 1 1 1 1 1 1 1 1 1 1 1 1 1 1 1 1 1 1 1 1 1 1 1 1 1 1 1 1 1 1 1 1 1 1 1 1 1 1 1 1 1 1 1 1 1 1 1 1 1 1 1 1 1 1 1 1 1]
  tag scope: T48_3891_3612217649251=global, T48_3892_3610730870102=global, T48_3892_3611023580993=global, T48_3892_3613942854876=global, T48_3893_3609891916485=global, T48_3893_3610244192181=global, T48_3893_3612454242394=global, T48_3893_3612747012868=global, T48_3893_3615779430918=global, T48_3894_3608822655727=global, T48_3894_3611613574610=global, T48_3894_3611965909889=global, T48_3894_3614288985102=global, T48_3894_3614581815160=global, T48_3895_3608040700638=global, T48_3895_3610542540102=global, T48_3895_3613446603152=global, T48_3895_3613798998014=global, T48_3896_3606833382123=global, T48_3896_3606918670479=global, T48_3896_3609758870847=global, T48_3896_3612373794894=global, T48_3897_3605989295953=global, T48_3897_3606015019504=global, T48_3897_3606086824096=global, T48_3897_3608549659415=global, T48_3897_3608634888187=global, T48_3897_3611588411472=global, T48_3898_3605169650195=global, T48_3898_3605259060634=global, T48_3898_3607703859078=global, T48_3898_3607729523045=global, T48_3898_3607801446804=global, T48_3898_3610377307123=global, T48_3898_3610462476312=global, T48_3899_3604565505514=global, T48_3899_3606882439570=global, T48_3899_3606971790426=global, T48_3899_3609529792620=global, T48_3899_3609555397004=global, T48_3899_3609627439929=global, T48_3900_3603717569929=global, T48_3900_3606276461556=global, T48_3900_3608706599362=global, T48_3900_3608795890634=global, T48_3901_3605426811804=global, T48_3901_3608098788014=global, T48_3902_3607247424096=global, T50_3987_3878106787188=global, T50_3988_3876876330955=global, T50_3988_3880102751020=global, T50_3989_3876391327041=global, T50_3989_3878870579351=global, T50_3989_3882216654453=global, T50_3990_3874595141290=global, T50_3990_3878383975249=global, T50_3990_3880982767347=global, T50_3991_3873544407857=global, T50_3991_3873985596037=global, T50_3991_3876585958812=global, T50_3991_3880494563057=global, T50_3992_3872553582024=global, T50_3992_3872653976445=global, T50_3992_3875533509943=global, T50_3992_3875974813371=global, T50_3992_3878694715935=global, T50_3993_3871661969078=global, T50_3993_3871819495433=global, T50_3993_3874540968673=global, T50_3993_3874641420718=global, T50_3993_3877640551629=global, T50_3993_3878081970306=global, T50_3994_3870891658078=global, T50_3994_3873647697914=global, T50_3994_3873805281894=global, T50_3994_3876646294922=global, T50_3994_3876746804592=global, T50_3995_3869893025229=global, T50_3995_3870141644180=global, T50_3995_3872875556229=global, T50_3995_3875751366351=global, T50_3995_3875909007955=global, T50_3996_3869045392576=global, T50_3996_3871875380816=global, T50_3996_3872123826894=global, T50_3996_3874977393980=global, T50_3997_3871025975102=global, T50_3997_3873975676004=global, T50_3997_3874223949208=global, T50_3998_3873124497229=global, T63_5456_6800259085392=global, T63_5457_6799545615796=global, T63_5458_6798975933185=global
  wires:
  v,i/1 -> Demux/1
  Demux/1 -> [T48_3896_3606918670479]
  Demux/2 -> [T48_3897_3608634888187]
  Demux/3 -> [T48_3898_3610462476312]
  Demux/4 -> [T50_3994_3870891658078]
  Demux/5 -> [T50_3995_3872875556229]
  Demux/6 -> [T50_3996_3874977393980]
  Demux/7 -> [T50_3995_3870141644180]
  Demux/8 -> [T50_3996_3872123826894]
  Demux/9 -> [T50_3997_3874223949208]
  Demux/10 -> [T50_3987_3878106787188]
  Demux/11 -> [T50_3988_3880102751020]
  Demux/12 -> [T50_3989_3882216654453]
  Demux/13 -> [T50_3988_3876876330955]
  Demux/14 -> [T50_3989_3878870579351]
  Demux/15 -> [T50_3990_3880982767347]
  Demux/16 -> [T48_3892_3610730870102]
  Demux/17 -> [T48_3893_3612454242394]
  Demux/18 -> [T48_3894_3614288985102]
  Demux/19 -> [T50_3990_3874595141290]
  Demux/20 -> [T50_3991_3876585958812]
  Demux/21 -> [T50_3992_3878694715935]
  Demux/22 -> [T50_3991_3873544407857]
  Demux/23 -> [T50_3992_3875533509943]
  Demux/24 -> [T50_3993_3877640551629]
  Demux/25 -> [T50_3992_3872553582024]
  Demux/26 -> [T50_3993_3874540968673]
  Demux/27 -> [T50_3994_3876646294922]
  Demux/28 -> [T48_3896_3606833382123]
  Demux/29 -> [T48_3897_3608549659415]
  Demux/30 -> [T48_3898_3610377307123]
  Demux/31 -> [T48_3897_3606015019504]
  Demux/32 -> [T48_3898_3607729523045]
  Demux/33 -> [T48_3899_3609555397004]
  Demux/34 -> [T48_3898_3605259060634]
  Demux/35 -> [T48_3899_3606971790426]
  Demux/36 -> [T48_3900_3608795890634]
  Demux/37 -> [T48_3899_3604565505514]
  Demux/38 -> [T48_3900_3606276461556]
  Demux/39 -> [T48_3901_3608098788014]
  Demux/40 -> [T48_3891_3612217649251]
  Demux/41 -> [T48_3892_3613942854876]
  Demux/42 -> [T48_3893_3615779430918]
  Demux/43 -> [T48_3892_3611023580993]
  Demux/44 -> [T48_3893_3612747012868]
  Demux/45 -> [T48_3894_3614581815160]
  Demux/46 -> [T48_3893_3609891916485]
  Demux/47 -> [T48_3894_3611613574610]
  Demux/48 -> [T48_3895_3613446603152]
  Demux/49 -> [T48_3894_3608822655727]
  Demux/50 -> [T48_3895_3610542540102]
  Demux/51 -> [T48_3896_3612373794894]
  Demux/52 -> [T50_3992_3872653976445]
  Demux/53 -> [T50_3993_3874641420718]
  Demux/54 -> [T50_3994_3876746804592]
  Demux/55 -> [T50_3993_3871661969078]
  Demux/56 -> [T50_3994_3873647697914]
  Demux/57 -> [T50_3995_3875751366351]
  Demux/58 -> [T48_3897_3605989295953]
  Demux/59 -> [T48_3898_3607703859078]
  Demux/60 -> [T48_3899_3609529792620]
  Demux/61 -> [T48_3898_3605169650195]
  Demux/62 -> [T48_3899_3606882439570]
  Demux/63 -> [T48_3900_3608706599362]
  Demux/64 -> [T50_3996_3869045392576]
  Demux/65 -> [T50_3997_3871025975102]
  Demux/66 -> [T50_3998_3873124497229]
  Demux/67 -> [T48_3900_3603717569929]
  Demux/68 -> [T48_3901_3605426811804]
  Demux/69 -> [T48_3902_3607247424096]
  Demux/70 -> [T50_3989_3876391327041]
  Demux/71 -> [T50_3990_3878383975249]
  Demux/72 -> [T50_3991_3880494563057]
  Demux/73 -> [T48_3893_3610244192181]
  Demux/74 -> [T48_3894_3611965909889]
  Demux/75 -> [T48_3895_3613798998014]
  Demux/76 -> [T50_3991_3873985596037]
  Demux/77 -> [T50_3992_3875974813371]
  Demux/78 -> [T50_3993_3878081970306]
  Demux/79 -> [T48_3895_3608040700638]
  Demux/80 -> [T48_3896_3609758870847]
  Demux/81 -> [T48_3897_3611588411472]
  Demux/82 -> [T50_3993_3871819495433]
  Demux/83 -> [T50_3994_3873805281894]
  Demux/84 -> [T50_3995_3875909007955]
  Demux/85 -> [T48_3897_3606086824096]
  Demux/86 -> [T48_3898_3607801446804]
  Demux/87 -> [T48_3899_3609627439929]
  Demux/88 -> [T50_3995_3869893025229]
  Demux/89 -> [T50_3996_3871875380816]
  Demux/90 -> [T50_3997_3873975676004]
  Demux/91 -> [T63_5456_6800259085392]
  Demux/92 -> [T63_5457_6799545615796]
  Demux/93 -> [T63_5458_6798975933185]

== system IEEE123_4subsystem/powergui/EquivalentModel9/Gates ==
  Mux : Mux  Inputs=[1 1 1]
  gates : Outport  VectorParamsAs1DForOutWhenUnconnected=off
  wires:
  Mux/1 -> gates/1
  [T49_3854_3555638165264] -> Mux/1
  [T49_3855_3558433039073] -> Mux/2
  [T49_3856_3561360060230] -> Mux/3

== system IEEE123_4subsystem/powergui/EquivalentModel9/Sources ==
  Mux : Mux  Inputs=[1 1 1 1 1 1 1 1 1 1 1 1 1 1 1 1 1 1 1 1 1 1 1 1 1 1 1 1 1 1 1 1 1 1 1]
  Mux_u : Mux  Inputs=[3 35]
  SwitchCurrents : Constant  Value=zeros(3,1)
  u : Outport  VectorParamsAs1DForOutWhenUnconnected=off
  wires:
  Mux_u/1 -> u/1
  SwitchCurrents/1 -> Mux_u/1
  Mux/1 -> Mux_u/2
  [T148_12731_30418452387025] -> Mux/1
  [T149_12782_30663996388773] -> Mux/2
  [T118_10142_19713599882240] -> Mux/3
  [T118_10144_19736951762083] -> Mux/4
  [T118_10146_19760975841562] -> Mux/5
  [T118_10148_19785672120675] -> Mux/6
  [T148_12733_30411660702877] -> Mux/7
  [T149_12784_30657204723230] -> Mux/8
  [T118_10144_19709202526933] -> Mux/9
  [T118_10146_19732548359945] -> Mux/10
  [T118_10148_19756566392592] -> Mux/11
  [T118_10150_19781256624873] -> Mux/12
  [T75_6128_8119493716371] -> Mux/13
  [T75_6129_8123585331178] -> Mux/14
  [T75_6130_8127883922252] -> Mux/15
  [T75_6129_8117491823106] -> Mux/16
  [T75_6130_8121581714011] -> Mux/17
  [T75_6131_8125878581182] -> Mux/18
  [T104_8898_14822538162015] -> Mux/19
  [T104_8899_14829093698812] -> Mux/20
  [T104_8900_14819929712314] -> Mux/21
  [T104_8901_14826481710679] -> Mux/22
  [T84_7400_12380292575747] -> Mux/23
  [T84_7401_12377637539587] -> Mux/24
  [T84_7402_12375090343665] -> Mux/25
  [T136_11679_24924668868749] -> Mux/26
  [T137_11730_25066490906578] -> Mux/27
  [T136_11681_24918803067887] -> Mux/28
  [T137_11732_25060624530635] -> Mux/29
  [T63_5076_5271644098914] -> Mux/30
  [T63_5077_5275502020138] -> Mux/31
  [T63_5078_5279538989299] -> Mux/32
  [T63_5077_5270525605105] -> Mux/33
  [T63_5078_5274381438295] -> Mux/34
  [T63_5079_5278416319421] -> Mux/35

== system IEEE123_4subsystem/powergui/EquivalentModel9/State-Space ==
  In1 : Inport
  In2 : Inport  Port=2
  ssn_sfun_sw1 : S-Function  FunctionName=ssn_sfun_v1  Parameters=9,0  SFunctionDeploymentMode=off  EnableBusSupport=off  SFcnStateName=MOV_segment59,xn_g1,xn_g2,xn_g3,xn_g4,xn_g5,MOV_segment59,MOV_segment59,MOV_segment59,MOV_segment59,MOV_segment59,MOV_segment59,MOV_segment59,MOV_segment59,MOV_segment59,MOV_segment59,MOV_segment59,MOV_segment59,MOV_segment59,MOV_segment59,MOV_segment59,MOV_segment59,MOV_segment59,MOV_segment59,MOV_segment59,MOV_segment59,MOV_segment59,MOV_segment59,MOV_segment59,MOV_segment59,MOV_segment59,MOV_segment59,MOV_segment59,MOV_segment59,MOV_segment59,MOV_segment59,MOV_segment59,MOV_segment59,MOV_segment59,MOV_segment59,MOV_segment59,MOV_segment59,MOV_segment59,MOV_segment59,MOV_segment59,MOV_segment59,MOV_segment59,MOV_segment59,MOV_segment59,MOV_segment59,MOV_segment59,MOV_segment59,MOV_segment59,MOV_segment59,MOV_segment59,MOV_segment59,MOV_segment59,MOV_segment59,MOV_segment59,MOV_segment59
      settings: SFcnIsStateOwnerBlock=on
  Out1 : Outport  VectorParamsAs1DForOutWhenUnconnected=off
  Out2 : Outport  Port=2  VectorParamsAs1DForOutWhenUnconnected=off
  tag scope: ssn_ext_sys_from_V_603x8dd7x9ebe8ae4d4e5=global, ssn_ext_sys_from_V_882xad52x737d12c533d7=global
  wires:
  ssn_sfun_sw1/2 -> Out2/1
  In2/1 -> ssn_sfun_sw1/2
  ssn_sfun_sw1/1 -> Out1/1
  In1/1 -> ssn_sfun_sw1/1
  [ssn_ext_sys_goto_Hist_882xad52x737d12c533d7] -> ssn_sfun_sw1/3
  [ssn_ext_sys_goto_Y_882xad52x737d12c533d7] -> ssn_sfun_sw1/4
  ssn_sfun_sw1/3 -> [ssn_ext_sys_from_V_882xad52x737d12c533d7]
  [ssn_ext_sys_goto_Hist_603x8dd7x9ebe8ae4d4e5] -> ssn_sfun_sw1/5
  [ssn_ext_sys_goto_Y_603x8dd7x9ebe8ae4d4e5] -> ssn_sfun_sw1/6
  ssn_sfun_sw1/4 -> [ssn_ext_sys_from_V_603x8dd7x9ebe8ae4d4e5]

== system IEEE123_4subsystem/powergui/EquivalentModel9/Status ==
  status : Inport
  Demux : Demux  Outputs=[1 1 1]
  tag scope: T51_4089_4363536697184=global, T51_4090_4365763736408=global, T51_4091_4368117740729=global
  wires:
  status/1 -> Demux/1
  Demux/1 -> [T51_4089_4363536697184]
  Demux/2 -> [T51_4090_4365763736408]
  Demux/3 -> [T51_4091_4368117740729]
